simulink model "lab1mod"  (Simulink 7.9)
settings: Solver=ode45  StartTime=0.0  StopTime=20.0  RelTol=1e-3
values from neighbouring files (symbols this model uses):
  alpha = 2*sqrt(c*M)    [lab1.m]    (also in lab1_simul.m = 500)
  c = 400    [lab1.m]    (also in lab1_simul.m)
  F = 1000    [lab1.m]    (also in lab1_simul.m)
  M = 1000    [lab1.m]    (also in lab1_simul.m)
settings Model: Creator=student  LastModifiedBy=student

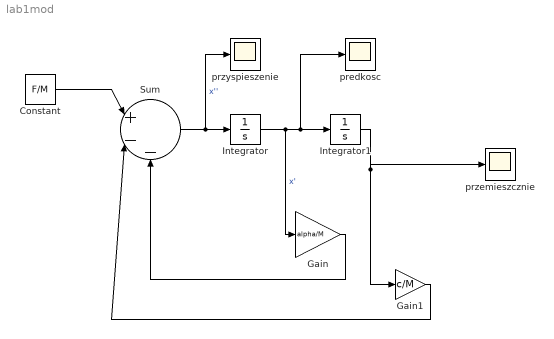
== system lab1mod ==
  Constant : Constant  Value=F/M
  Gain : Gain  Gain=alpha/M
  Gain1 : Gain  Gain=c/M
  Integrator : Integrator
  Integrator1 : Integrator
  Sum : Sum  Inputs=|+--
  predkosc : Scope
  przemieszcznie : Scope
      settings: SaveName=ScopeData2
  przyspieszenie : Scope
  wires:
  Sum/1 -> Integrator/1, przyspieszenie/1  "x''"
  Integrator/1 -> Gain/1, Integrator1/1, predkosc/1  "x'"
  Gain/1 -> Sum/3
  Integrator1/1 -> Gain1/1, przemieszcznie/1
  Gain1/1 -> Sum/2
  Constant/1 -> Sum/1
